simulink model "remoteMicrogrid"  (R2023a)
settings: Solver=FixedStepDiscrete  StartTime=0.0  StopTime=8  FixedStep=Ts  RelTol=1e-3
PreLoadFcn:
  | remoteMicrogridInputData
undefined symbols (not defined in the file): BESS, ControlRoom, DiscIntNeverNeededParam, Grid, Load, Machine, Microgrid, PV, T_on, Ts
libraries: ee_lib x46, eeGeneralControl x35, nesl_utility_internal x25, simulink x24, nesl_utility x20, fl_lib x17, slpidlib x12, eeTransforms x5, eeRmsMeasurement x4, eeTotalHarmonicDistorsion x4, eeSinusoidalMeasurement x3, batteryecm_lib x2
(part 1 of 5)
CloseFcn:
  | try,close(h1_remote_microgrid),end
  | clear h1_remote_microgrid
  | try,close(h2_remote_microgrid),end
  | clear h2_remote_microgrid
  | try,close(h2a_remote_microgrid),end
  | clear h2a_remote_microgrid
  | try,close(h3_remote_microgrid),end
  | clear h3_remote_microgrid
  | try,close(h4_remote_microgrid),end
  | clear h4_remote_microgrid
  | clear BESS closedLoop controller currentLoopPole
  | clear fsw_V geometricMean grid Grid inverter KI_PVPLL
  | clear KP_PVPLL logsout_remote_microgrid
  | clear Microgrid PrimaryreactancePV PrimaryresistancePV
  | clear remainingPowerPerString SecondaryreactancePV
  | clear SecondaryresistancePV sensor simlog_remote_microgrid
  | clear simulation solarPanel solarPlant TransformerPrimaryVoltagePV
  | clear TransformerRatingPV TransformerSecondaryVoltagePV
  | clear Ts Ts_V Solar logsout_remote_microgrid simlog_remote_microgrid
  | clear caseNum ControlRoom Load Machine tStart tStop
  | clear transformer_lv transformer_hv transformer_VA
  | clear transformer_winding_resistance transformer_winding_lekage_reactance
  | clear transformer_zero_sequence_reactance I_max_pu Vdc C L KV_base_new
  | clear MVA_base_new z_base n_series_cell_panel n_parallel_strings_panel
  | clear n_series_panels_per_string n_parallel_strings t_sensor
  | clear Kp_ic Ki_ic Kd Kp_v Ki_v Kd_v Vdc_base
  | clear Kp_pll Ki_pll
  | clear diode_saturation_current solar_generated_current_AM
  | clear quality_factor_i quality_factor_j Solar_cell.series_resistance
  | clear parallel_resistance temp_cofficient Eg temparature_exponent_Is1
  | clear temparature_exponent_Is2 temparature_exponent_Rs temparature_exponent_Rp
  | clear measurement_temperature device_temperature
  | clear PV Solar_cell T_on
  | clear BESSCost1 BESSCost2 BESSCost3 BESSCost4 BESSCost5 BESSKVAs1 BESSKVAs2
  | clear BESSKVAs3 BESSKVAs4 BESSKVAs5 Diesel_cost_s1 Diesel_cost_s1_yr Diesel_cost_s2
  | clear Diesel_cost_s2_yr Diesel_cost_s3 Diesel_cost_s3_yr Diesel_cost_s4 Diesel_cost_s4_yr
  | clear Diesel_cost_s5 Diesel_cost_s5_yr diesel_litre_USD Diesel_loading_100percent
  | clear Diesel_loading_25percent Diesel_loading_50percent Diesel_loading_75percent
  | clear Diesel_s1 Diesel_s2 Diesel_s3 Diesel_s4 Diesel_s5 DieselKVAs1 DieselKVAs2
  | clear DieselKVAs3 DieselKVAs4 DieselKVAs5 frequencyLimit logsout1 logsout2 logsout3
  | clear logsout4 logsout_activeloss1 logsout_activeloss2 logsout_activeloss3
  | clear logsout_activeloss4 logsout_freqmax1 logsout_freqmax2 logsout_freqmax3
  | clear logsout_freqmax4 logsout_freqmin1 logsout_freqmin2 logsout_freqmin3 logsout_freqmin4
  | clear logsout_LoadTHD1 logsout_LoadTHD2 logsout_LoadTHD3 logsout_LoadTHD4
  | clear logsout_MaxLoadVoltage1 logsout_MaxLoadVoltage2 logsout_MaxLoadVoltage3
  | clear logsout_MaxLoadVoltage4 logsout_MinLoadVoltage1 logsout_MinLoadVoltage2
  | clear logsout_MinLoadVoltage3 logsout_MinLoadVoltage4 logsout_PCCTHD1 logsout_PCCTHD2
  | clear logsout_PCCTHD3 logsout_PCCTHD4 logsout_reactiveloss1 logsout_reactiveloss2
  | clear logsout_reactiveloss3 logsout_reactiveloss4 logsout_volmax1 logsout_volmax2
  | clear logsout_volmax3 logsout_volmax4 logsout_volmin1 logsout_volmin2 logsout_volmin3
  | clear logsout_volmin4 Micorgrid TotalCost1 TotalCost2 TotalCost3 TotalCost4 TotalCost5
  | clear voltageLimit xlim xticks
Description:
  | Copyright 2022 - 2023 The MathWorks, Inc.
settings Model: Creator=The MathWorks, Inc.  LastModifiedBy=skota
settings SolverCC: AlgebraicLoopSolver=TrustRegion
settings DataIOCC: SaveOutput=off  SaveTime=off  ReturnWorkspaceOutputs=off  SignalLoggingName=logsout_remote_microgrid  OutputTimes=[0:1.1*3*Voc/(1*2000):1.1*3*Voc/1]
settings OptimizationCC: ReuseModelBlockBuffer=off
settings DebuggingCC: UnconnectedInputMsg=warning  UnconnectedOutputMsg=warning  UnconnectedLineMsg=warning  StateNameClashWarn=warning  ArithmeticOperatorsInVariantConditions=warning
settings HardwareCC: ProdBitPerPointer=32  ProdBitPerSizeT=32  ProdBitPerPtrDiffT=32  ProdWordSize=32  ProdHWDeviceType=Intel->x86-32 (Windows32)
settings ModelReferenceCC: EnableRefExpFcnMdlSchedulingChecks=on  PropagateSignalLabelsOutOfModel=off
settings SFSimCC: CustomCodeUndefinedFunction=UseInterfaceOnly
settings RTWCC: DLArmComputeVersion=19.05
settings CodeAppCC: StateflowObjectComments=on
settings SimscapeCC: SimscapeNominalValues="[{\"value\":\"1\",\"unit\":\"A\"},{\"value\":\"1\",\"unit\":\"bar\"},{\"value\":\"1\",\"unit\":\"cm^2\"},{\"value\":\"1\",\"unit\":\"cm^3/s\"},{\"value\":\"1\",\"unit\":\"kJ/kg\"},{\"value\":\"1\",\"unit\":\"kW\"},{\"value\":\"1\",\"unit\":\"l\"},{\"value\":\"1\",\"unit\":\"N\"},{\"value\":\"1\",\"unit\":\"N*m\"},{\"value\":\"1e3\",\"unit\":\"V\"}]"  SimscapeLogType=all  SimscapeLogSimulationStatistics=on  SimscapeLogName=simlog_remote_microgrid  SimscapeLogLimitData=off

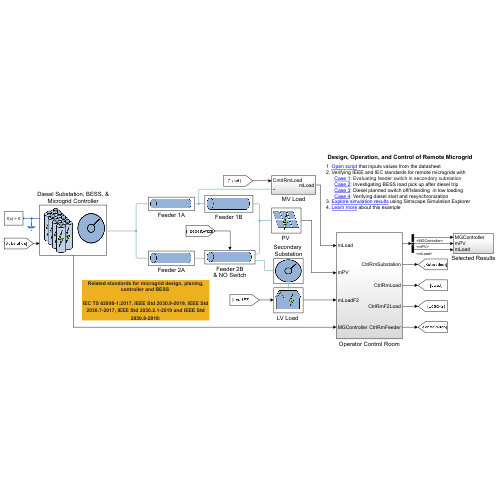
[thumbnail: Simulink's stored preview of the top-level diagram]
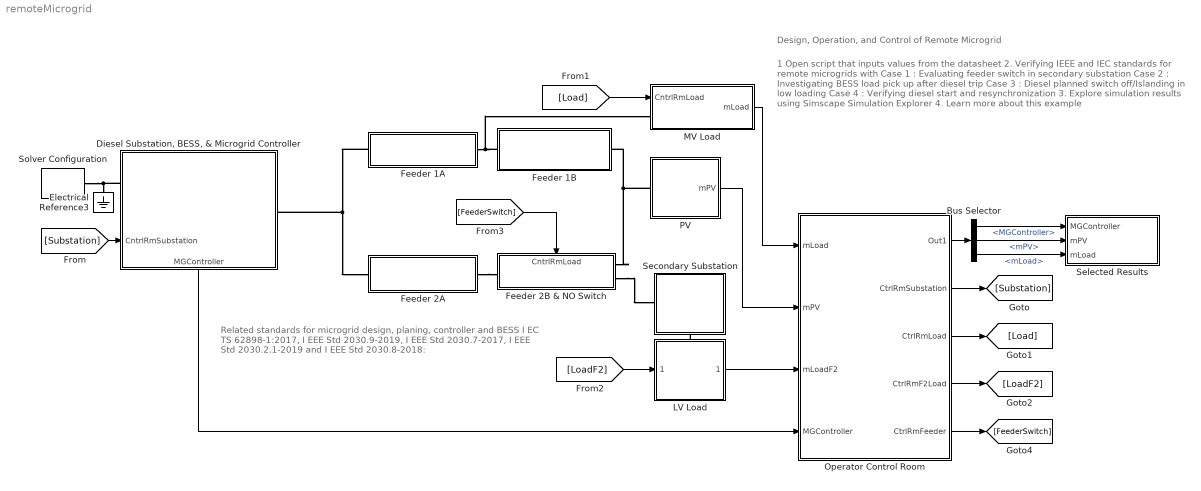
== system remoteMicrogrid ==
  note: Related standards for microgrid design, planing, controller and BESS
      | I EC TS 62898-1:2017, I EEE Std 2030.9-2019, I EEE Std 2030.7-2017, I EEE Std 2030.2.1-2019 and I EEE Std 2030.8-2018:
  note: Design, Operation, and Control of Remote Microgrid
  note: 1 Open script that inputs values from the datasheet
      | 2. Verifying IEEE and IEC standards for remote microgrids with
      | Case 1 : Evaluating feeder switch in secondary substation
      | Case 2 : Investigating BESS load pick up after diesel trip
      | Case 3 : Diesel planned switch off/Islanding in low loading
      | Case 4 : Verifying diesel start and resynchronization
      | 3. Explore simulation results using Simscape Simulation Explorer
      | 4. Learn more about this example
  Bus Selector : BusSelector  OutputSignals=MGController,mPV,mLoad
  "Diesel Substation, BESS, & Microgrid Controller" : Subsystem
      settings: PortSchema="{\"entries\":[{\"content\":{\"sides\":[{\"content\":{\"connectorIds\":[\"LConn1\",\"In1\"]},\"type\":\"ConnectorPlacement.EquallySpacedRectSide\",\"uuid\":\"34af2ba0-e960-4f27-b72f-7309cde5bec1\"},{\"content\":{\"connectorIds\":[\"RConn1\"],\"side\":\"RIGHT\"},\"type\":\"ConnectorPlacement.EquallySpacedRectSide\",\"uuid\":\"58e91d81-71e9-481c-b1fd-5cc7b2cbdd18\"},{\"content\":{\"connectorIds\":[],\"side\":\"TOP\"},\"type\":\"ConnectorPlacement.EquallySpacedRectSide\",\"uuid\":\"32e6dd42-e4bf-406e-9b62-7b4d690f744b\"},{\"content\":{\"connectorIds\":[\"Out1\"],\"side\":\"BOTTOM\"},\"type\":\"ConnectorPlacement.EquallySpacedRectSide\",\"uuid\":\"17a24731-c833-4ec2-b0a2-39897b42a00f\"}]},\"type\":\"ConnectorPlacement.EquallySpacedConnector\",\"uuid\":\"86c228e9-32f4-4f18-a8a0-642828fccfbb\"}],\"packageUris\":[\"http://schema.mathworks.com/mf0/Connector/R2020b\"],\"version\":\"1.0\"}"
      mask Display: image('$imagefile'); % Use "Edit Image" on toolstrip to change.
  Electrical Reference3 : fl_lib/Electrical/Electrical Elements/Electrical Reference
  Feeder 1A : Subsystem
      mask Display: image('$imagefile'); % Use "Edit Image" on toolstrip to change.
  Feeder 1B : Subsystem
      mask Display: image('$imagefile'); % Use "Edit Image" on toolstrip to change.
  Feeder 2A : Subsystem
      mask Display: image('$imagefile'); % Use "Edit Image" on toolstrip to change.
  Feeder 2B & NO Switch : Subsystem
      settings: PortSchema="{\"entries\":[{\"content\":{\"sides\":[{\"content\":{\"connectorIds\":[\"LConn1\"]},\"type\":\"ConnectorPlacement.EquallySpacedRectSide\",\"uuid\":\"1b47678a-34eb-4830-a1d8-8584b0b3d2f8\"},{\"content\":{\"connectorIds\":[\"RConn1\",\"RConn2\"],\"side\":\"RIGHT\"},\"type\":\"ConnectorPlacement.EquallySpacedRectSide\",\"uuid\":\"1e19bb0d-7be0-4a53-b6f3-f72359312777\"},{\"content\":{\"connectorIds\":[\"In1\"],\"side\":\"TOP\"},\"type\":\"ConnectorPlacement.EquallySpacedRectSide\",\"uuid\":\"6a5adcb0-1c8a-4af3-8ce7-b7b52f7f2199\"}]},\"type\":\"ConnectorPlacement.EquallySpacedConnector\",\"uuid\":\"0f133d9b-a960-48f9-af57-ff4de668ee2e\"}],\"packageUris\":[\"http://schema.mathworks.com/mf0/Connector/R2020b\"],\"version\":\"1.0\"}"
      mask Display: image('$imagefile'); % Use "Edit Image" on toolstrip to change.
  "LV Load " : Subsystem
      settings: PortSchema="{\"entries\":[{\"content\":{\"sides\":[{\"content\":{\"connectorIds\":[\"In1\"]},\"type\":\"ConnectorPlacement.EquallySpacedRectSide\",\"uuid\":\"cc4763ec-9449-4f2d-b299-5261ad2f5cfe\"},{\"content\":{\"connectorIds\":[\"Out1\"],\"side\":\"RIGHT\"},\"type\":\"ConnectorPlacement.EquallySpacedRectSide\",\"uuid\":\"9da329b8-70a1-4faf-a44a-2cf8be9addec\"},{\"content\":{\"connectorIds\":[\"LConn1\"],\"side\":\"TOP\"},\"type\":\"ConnectorPlacement.EquallySpacedRectSide\",\"uuid\":\"c4abe44e-3291-4dff-9d7a-9215b8ef2faf\"}]},\"type\":\"ConnectorPlacement.EquallySpacedConnector\",\"uuid\":\"e73dbaae-f88f-4a7a-af91-27ace77c935e\"}],\"packageUris\":[\"http://schema.mathworks.com/mf0/Connector/R2020b\"],\"version\":\"1.0\"}"
      mask Display: image('$imagefile'); % Use "Edit Image" on toolstrip to change.
  MV Load : Subsystem
  Operator Control Room : Subsystem
      settings: PortSchema="{\"entries\":[{\"content\":{\"sides\":[{\"content\":{\"connectorIds\":[\"Out1\",\"Out2\",\"Out3\",\"Out4\",\"Out5\"]},\"type\":\"ConnectorPlacement.EquallySpacedRectSide\",\"uuid\":\"36e3c748-e70d-4376-8c54-bee35c2cf55e\"},{\"content\":{\"connectorIds\":[\"In1\",\"In2\",\"In3\",\"In4\"],\"side\":\"RIGHT\"},\"type\":\"ConnectorPlacement.EquallySpacedRectSide\",\"uuid\":\"3af4b9ea-3351-4c6c-90c1-760bf6d2a862\"},{\"content\":{\"connectorIds\":[],\"side\":\"TOP\"},\"type\":\"ConnectorPlacement.EquallySpacedRectSide\",\"uuid\":\"c84439f5-3dbb-4f33-afb8-95498296d6fa\"}]},\"type\":\"ConnectorPlacement.EquallySpacedConnector\",\"uuid\":\"cafa6b3a-2446-4c45-9268-4fc6f6c2350c\"}],\"packageUris\":[\"http://schema.mathworks.com/mf0/Connector/R2020b\"],\"version\":\"1.0\"}"
  "PV " : Subsystem
      mask Display: image('$imagefile'); % Use "Edit Image" on toolstrip to change.
  Secondary Substation : Subsystem
      settings: PortSchema="{\"entries\":[{\"content\":{\"sides\":[{\"content\":{\"connectorIds\":[\"LConn1\"]},\"type\":\"ConnectorPlacement.EquallySpacedRectSide\",\"uuid\":\"e00206b4-f52b-4711-97fc-4887ea8823c3\"},{\"content\":{\"connectorIds\":[],\"side\":\"RIGHT\"},\"type\":\"ConnectorPlacement.EquallySpacedRectSide\",\"uuid\":\"71e01694-379b-4552-8103-40d657e486e9\"},{\"content\":{\"connectorIds\":[],\"side\":\"TOP\"},\"type\":\"ConnectorPlacement.EquallySpacedRectSide\",\"uuid\":\"04395bce-e736-431c-9f74-8350dc9d2f2b\"},{\"content\":{\"connectorIds\":[\"RConn1\"],\"side\":\"BOTTOM\"},\"type\":\"ConnectorPlacement.EquallySpacedRectSide\",\"uuid\":\"4a9ed1b9-5a03-4ea2-8ce4-b63f4eba4172\"}]},\"type\":\"ConnectorPlacement.EquallySpacedConnector\",\"uuid\":\"55927287-d52f-4d79-aceb-3e97c7a13d06\"}],\"packageUris\":[\"http://schema.mathworks.com/mf0/Connector/R2020b\"],\"version\":\"1.0\"}"
      mask Display: image('$imagefile'); % Use "Edit Image" on toolstrip to change.
  Selected Results : Subsystem
  Solver Configuration : nesl_utility_internal/Solver Configuration  PhysicalDomain=network_engine_domain  SubClassName=solver  LeftPortType=input  RightPortType=generic  Tones=[]  Harmonics=[]  SimulateNoise=off  Profile=off  UseLocalSampling=off  EnableSwitchedLinearOptims=on  FrequencyDomain=off  UseCCode=off  RelTol=0.001  AbsTol=1e-06  MinStep=1e-09  ToWorkspace=off  RevertToSquareIcSolve=off  NumHomotopyIterations=100  PhasorMode=off  PhasorModeNumHarmonics=1  ConsistencySolver=NEWTON_FTOL  IndexReductionMethod=DerivativeReplacement  DoDC=off  ResidualTolerance=1e-07  ConsistencyTolSource=GLOBAL  ConsistencyAbsTol=0.001  ConsistencyRelTol=0.001  ConsistencyTolFactor=0.001  UseLocalSolver=on  LocalSolverChoice=NE_BACKWARD_EULER_ADVANCER  ResolveIndetEquations=on  FunctionEvalNumThread=1  LocalSolverSampleTime=Ts  DoFixedCost=on  MaxNonlinIter=3  MaxModeIter=2  ComputeImpulses=off  ImpulseIterations=1  LinearAlgebra=auto  LinearAlgebraNumThread=0  EquationFormulation=NE_TIME_EF  DelaysMemoryBudget=1024  AutomaticFiltering=off  FilteringTimeConstant=0.001  PartitionStorageMethod=AS_NEEDED  PartitionMemoryBudget=1024  PartitionMethod=FAST
  wires:
  Operator Control Room/2(CtrlRmSubstation) -> [Substation]
  Bus Selector/1 -> Selected Results/1(MGController)  "<MGController>"
  Bus Selector/2 -> Selected Results/2(mPV)  "<mPV>"
  Bus Selector/3 -> Selected Results/3(mLoad)  "<mLoad>"
  Operator Control Room/1(Out1) -> Bus Selector/1
  [Substation] -> "Diesel Substation, BESS, & Microgrid Controller"/1(CntrlRmSubstation)
  "LV Load "/1(mLoadF2) -> Operator Control Room/3(mLoadF2)
  MV Load/1(mLoad) -> Operator Control Room/1(mLoad)
  "Diesel Substation, BESS, & Microgrid Controller"/1(MGController) -> Operator Control Room/4(MGController)
  [Load] -> MV Load/1(CntrlRmLoad)
  [LoadF2] -> "LV Load "/1(CtrlRmF2Load)
  Operator Control Room/3(CtrlRmLoad) -> [Load]
  Operator Control Room/4(CtrlRmF2Load) -> [LoadF2]
  Operator Control Room/5(CtrlRmFeeder) -> [FeederSwitch]
  "PV "/1(mPV) -> Operator Control Room/2(mPV)
  [FeederSwitch] -> Feeder 2B & NO Switch/1(CntrlRmLoad)
  connections:
  "LV Load "/LConn1 -- Secondary Substation/RConn1
  Solver Configuration/RConn1 -- Electrical Reference3/LConn1 -- "Diesel Substation, BESS, & Microgrid Controller"/LConn1
  "PV "/LConn1 -- Feeder 2B & NO Switch/RConn1 -- Feeder 1B/RConn1
  Feeder 1A/RConn1 -- MV Load/LConn1 -- Feeder 1B/LConn1
  Feeder 1A/LConn1 -- Feeder 2A/LConn1 -- "Diesel Substation, BESS, & Microgrid Controller"/RConn1
  Feeder 2B & NO Switch/RConn2 -- Secondary Substation/LConn1
  Feeder 2A/RConn1 -- Feeder 2B & NO Switch/LConn1

== system remoteMicrogrid/Diesel Substation, BESS, & Microgrid Controller ==
  CntrlRmSubstation : Inport
  BESS and Controller : Subsystem
  Bus Creator : BusCreator  Inputs=3
  CntrlRmSubstation1 : InportShadow
  Diesel Generator : Subsystem
  Microgrid Controller : Subsystem
      settings: PortSchema="{\"entries\":[{\"content\":{\"sides\":[{\"content\":{\"connectorIds\":[\"In1\",\"In2\",\"In3\"]},\"type\":\"ConnectorPlacement.EquallySpacedRectSide\",\"uuid\":\"5a677e32-2413-4856-9683-7f083fbde1c7\"},{\"content\":{\"connectorIds\":[\"RConn1\",\"Out1\",\"Out2\"],\"side\":\"RIGHT\"},\"type\":\"ConnectorPlacement.EquallySpacedRectSide\",\"uuid\":\"93a85587-a429-4479-a8cb-2de590d95871\"},{\"content\":{\"connectorIds\":[],\"side\":\"TOP\"},\"type\":\"ConnectorPlacement.EquallySpacedRectSide\",\"uuid\":\"c42d9fd8-4416-4e89-82a5-0d6c34ce0f8c\"}]},\"type\":\"ConnectorPlacement.EquallySpacedConnector\",\"uuid\":\"0378cbf3-df98-42a2-a108-9ea24e13e829\"}],\"packageUris\":[\"http://schema.mathworks.com/mf0/Connector/R2020b\"],\"version\":\"1.0\"}"
  PCC Measurements and PCC Breaker : Subsystem
      settings: PortSchema="{\"entries\":[{\"content\":{\"sides\":[{\"content\":{\"connectorIds\":[\"LConn1\"]},\"type\":\"ConnectorPlacement.EquallySpacedRectSide\",\"uuid\":\"04177ba8-e6a4-4482-9e4e-86e01b546ca8\"},{\"content\":{\"connectorIds\":[\"RConn1\",\"RConn2\",\"Out1\"],\"side\":\"RIGHT\"},\"type\":\"ConnectorPlacement.EquallySpacedRectSide\",\"uuid\":\"b1feeba7-b9e0-4dc8-9251-9fa4e491a467\"},{\"content\":{\"connectorIds\":[],\"side\":\"TOP\"},\"type\":\"ConnectorPlacement.EquallySpacedRectSide\",\"uuid\":\"26b7aa1a-5290-4eee-bcf5-b11865d5ca2e\"}]},\"type\":\"ConnectorPlacement.EquallySpacedConnector\",\"uuid\":\"5841c04a-e0b1-4fd8-9efd-d8c83177b337\"}],\"packageUris\":[\"http://schema.mathworks.com/mf0/Connector/R2020b\"],\"version\":\"1.0\"}"
  Transformer and Disconnectors : Subsystem
  ref : PMIOPort  Side=Left
  "~ " : PMIOPort  Port=2  Side=Right
  MGController : Outport
  wires:
  PCC Measurements and PCC Breaker/1(" mPCC") -> Microgrid Controller/1("mPCC ")
  CntrlRmSubstation/1 -> BESS and Controller/2(CntrlRmSubstation)
  BESS and Controller/1(mBESS) -> Microgrid Controller/3(BESS), Bus Creator/3  "BESS"
  Bus Creator/1 -> MGController/1
  Microgrid Controller/1(BESSRef) -> [BESSref], Bus Creator/1  "References and BRK"
  CntrlRmSubstation1/1 -> Microgrid Controller/2(CntrlRmSubstation)
  [BESSref] -> BESS and Controller/1(BESSRef)
  Microgrid Controller/2(MGController) -> Bus Creator/2  "Controller"
  connections:
  Microgrid Controller/RConn1 -- PCC Measurements and PCC Breaker/RConn2
  "~ "/RConn1 -- PCC Measurements and PCC Breaker/RConn1 -- BESS and Controller/RConn1
  Transformer and Disconnectors/RConn1 -- PCC Measurements and PCC Breaker/LConn1
  Transformer and Disconnectors/LConn1 -- Diesel Generator/RConn1
  ref/RConn1 -- Diesel Generator/LConn1

== system remoteMicrogrid/Feeder 1A ==
  "Line X/R=1.44 " : ee_lib/Passive/RLC Assemblies/RLC (Three-Phase)  component_structure=ee.enum.rlc.structure.SeriesRL  R=Microgrid.R_line Ohm  L=Microgrid.L_line H  C=1 F  R_parasitic=1e-6 Ohm  G_parasitic=1e-5 1/Ohm  IL_specify=on  IL_priority=High  IL=[0, 0, 0] A  IL_nominal_specify=off  IL_nominal_unit=A  IL_nominal_value=1  VC_specify=on  VC_priority=High  VC=[0, 0, 0] V  VC_nominal_specify=off  VC_nominal_unit=V  VC_nominal_value=1
      settings: InternalSimscapePortConfiguration="{\"Bottom\":[],\"Left\":[{\"id\":\"N1\",\"label\":\"~1\",\"type\":\"foundation.electrical.three_phase\"}],\"Right\":[{\"id\":\"N2\",\"label\":\"~2\",\"type\":\"foundation.electrical.three_phase\"}],\"Top\":[]}"
  Conn1 : PMIOPort  Side=Right
  Conn2 : PMIOPort  Port=2  Side=Left
  connections:
  "Line X/R=1.44 "/RConn1 -- Conn1/RConn1
  "Line X/R=1.44 "/LConn1 -- Conn2/RConn1

== system remoteMicrogrid/Feeder 1B ==
  Line X/R=1.44 : ee_lib/Passive/RLC Assemblies/RLC (Three-Phase)  component_structure=ee.enum.rlc.structure.SeriesRL  R=Microgrid.R_line Ohm  L=Microgrid.L_line H  C=1 F  R_parasitic=1e-6 Ohm  G_parasitic=1e-5 1/Ohm  IL_specify=on  IL_priority=High  IL=[0, 0, 0] A  IL_nominal_specify=off  IL_nominal_unit=A  IL_nominal_value=1  VC_specify=on  VC_priority=High  VC=[0, 0, 0] V  VC_nominal_specify=off  VC_nominal_unit=V  VC_nominal_value=1
      settings: InternalSimscapePortConfiguration="{\"Bottom\":[],\"Left\":[{\"id\":\"N1\",\"label\":\"~1\",\"type\":\"foundation.electrical.three_phase\"}],\"Right\":[{\"id\":\"N2\",\"label\":\"~2\",\"type\":\"foundation.electrical.three_phase\"}],\"Top\":[]}"
  Conn1 : PMIOPort  Side=Left
  Conn2 : PMIOPort  Port=2  Side=Right
  connections:
  Line X/R=1.44/LConn1 -- Conn1/RConn1
  Conn2/RConn1 -- Line X/R=1.44/RConn1

== system remoteMicrogrid/Feeder 2A ==
  "Line X/R=1.44  " : ee_lib/Passive/RLC Assemblies/RLC (Three-Phase)  component_structure=ee.enum.rlc.structure.SeriesRL  R=Microgrid.R_line Ohm  L=Microgrid.L_line H  C=1 F  R_parasitic=1e-6 Ohm  G_parasitic=1e-5 1/Ohm  IL_specify=on  IL_priority=High  IL=[0, 0, 0] A  IL_nominal_specify=off  IL_nominal_unit=A  IL_nominal_value=1  VC_specify=on  VC_priority=High  VC=[0, 0, 0] V  VC_nominal_specify=off  VC_nominal_unit=V  VC_nominal_value=1
      settings: InternalSimscapePortConfiguration="{\"Bottom\":[],\"Left\":[{\"id\":\"N1\",\"label\":\"~1\",\"type\":\"foundation.electrical.three_phase\"}],\"Right\":[{\"id\":\"N2\",\"label\":\"~2\",\"type\":\"foundation.electrical.three_phase\"}],\"Top\":[]}"
  Conn2 : PMIOPort  Side=Left
  Conn1 : PMIOPort  Port=2  Side=Right
  connections:
  Conn2/RConn1 -- "Line X/R=1.44  "/LConn1
  Conn1/RConn1 -- "Line X/R=1.44  "/RConn1

== system remoteMicrogrid/Feeder 2B & NO Switch ==
  Bus Element In2 : Inport  PortName=CntrlRmLoad  Element=FeederSwitch
  " Line X/R=1.44 " : ee_lib/Passive/RLC Assemblies/RLC (Three-Phase)  component_structure=ee.enum.rlc.structure.SeriesRL  R=Microgrid.R_line Ohm  L=Microgrid.L_line H  C=1 F  R_parasitic=1e-6 Ohm  G_parasitic=1e-5 1/Ohm  IL_specify=on  IL_priority=High  IL=[0, 0, 0] A  IL_nominal_specify=off  IL_nominal_unit=A  IL_nominal_value=1  VC_specify=on  VC_priority=High  VC=[0, 0, 0] V  VC_nominal_specify=off  VC_nominal_unit=V  VC_nominal_value=1
      settings: InternalSimscapePortConfiguration="{\"Bottom\":[],\"Left\":[{\"id\":\"N1\",\"label\":\"~1\",\"type\":\"foundation.electrical.three_phase\"}],\"Right\":[{\"id\":\"N2\",\"label\":\"~2\",\"type\":\"foundation.electrical.three_phase\"}],\"Top\":[]}"
  " Line X/R=1.44 1" : ee_lib/Passive/RLC Assemblies/RLC (Three-Phase)  component_structure=ee.enum.rlc.structure.SeriesRL  R=Microgrid.R_line Ohm  L=Microgrid.L_line H  C=1 F  R_parasitic=1e-6 Ohm  G_parasitic=1e-5 1/Ohm  IL_specify=on  IL_priority=High  IL=[0, 0, 0] A  IL_nominal_specify=off  IL_nominal_unit=A  IL_nominal_value=1  VC_specify=on  VC_priority=High  VC=[0, 0, 0] V  VC_nominal_specify=off  VC_nominal_unit=V  VC_nominal_value=1
      settings: InternalSimscapePortConfiguration="{\"Bottom\":[],\"Left\":[{\"id\":\"N1\",\"label\":\"~1\",\"type\":\"foundation.electrical.three_phase\"}],\"Right\":[{\"id\":\"N2\",\"label\":\"~2\",\"type\":\"foundation.electrical.three_phase\"}],\"Top\":[]}"
  Circuit Breaker (Three-Phase) : ee_lib/Switches & Breakers/Circuit Breaker (Three-Phase)  R_closed=0.001 Ohm  G_open=1e-6 1/Ohm  threshold=0.5 V  breaker_behavior=ee.enum.switches.breakerBehavior.zeroCrossingDisable
      settings: InternalSimscapePortConfiguration="{\"Bottom\":[],\"Left\":[{\"id\":\"vT\",\"label\":\"vT\",\"type\":\"input\"},{\"id\":\"N1\",\"label\":\"~1\",\"type\":\"foundation.electrical.three_phase\"}],\"Right\":[{\"id\":\"N2\",\"label\":\"~2\",\"type\":\"foundation.electrical.three_phase\"}],\"Top\":[]}"
  Circuit Breaker (Three-Phase)1 : ee_lib/Switches & Breakers/Circuit Breaker (Three-Phase)  R_closed=0.001 Ohm  G_open=1e-6 1/Ohm  threshold=0.5 V  breaker_behavior=ee.enum.switches.breakerBehavior.zeroCrossingDisable
      settings: InternalSimscapePortConfiguration="{\"Bottom\":[],\"Left\":[{\"id\":\"vT\",\"label\":\"vT\",\"type\":\"input\"},{\"id\":\"N1\",\"label\":\"~1\",\"type\":\"foundation.electrical.three_phase\"}],\"Right\":[{\"id\":\"N2\",\"label\":\"~2\",\"type\":\"foundation.electrical.three_phase\"}],\"Top\":[]}"
  Subsystem : Subsystem
  Conn2 : PMIOPort  Side=Left
  Feeder1BRK : PMIOPort  Port=2  Side=Right
  Feeder2BRK : PMIOPort  Port=3  Side=Right
  wires:
  Bus Element In2/1 -> Subsystem/1(ControlRoom)
  connections:
  Circuit Breaker (Three-Phase)/LConn2 -- " Line X/R=1.44 "/RConn1
  " Line X/R=1.44 1"/LConn1 -- Feeder2BRK/RConn1
  Conn2/RConn1 -- Circuit Breaker (Three-Phase)1/LConn2
  Subsystem/RConn1 -- Circuit Breaker (Three-Phase)/LConn1
  " Line X/R=1.44 "/LConn1 -- " Line X/R=1.44 1"/RConn1 -- Circuit Breaker (Three-Phase)1/RConn1
  Subsystem/RConn2 -- Circuit Breaker (Three-Phase)1/LConn1
  Circuit Breaker (Three-Phase)/RConn1 -- Feeder1BRK/RConn1

== system remoteMicrogrid/LV Load  ==
  Bus Element In3 : Inport  PortName=CtrlRmF2Load  Element=Load2BControl
  Bus Element In1 : Inport  PortName=CtrlRmF2Load  Element=Load2AControl
  Circuit Breaker (Three-Phase)1 : ee_lib/Switches & Breakers/Circuit Breaker (Three-Phase)  R_closed=0.001 Ohm  G_open=1e-6 1/Ohm  threshold=0.5 V  breaker_behavior=ee.enum.switches.breakerBehavior.zeroCrossingEnable
      settings: InternalSimscapePortConfiguration="{\"Bottom\":[],\"Left\":[{\"id\":\"vT\",\"label\":\"vT\",\"type\":\"input\"},{\"id\":\"N1\",\"label\":\"~1\",\"type\":\"foundation.electrical.three_phase\"}],\"Right\":[{\"id\":\"N2\",\"label\":\"~2\",\"type\":\"foundation.electrical.three_phase\"}],\"Top\":[]}"
  Circuit Breaker (Three-Phase)2 : ee_lib/Switches & Breakers/Circuit Breaker (Three-Phase)  R_closed=0.001 Ohm  G_open=1e-6 1/Ohm  threshold=0.5 V  breaker_behavior=ee.enum.switches.breakerBehavior.zeroCrossingEnable
      settings: InternalSimscapePortConfiguration="{\"Bottom\":[],\"Left\":[{\"id\":\"vT\",\"label\":\"vT\",\"type\":\"input\"},{\"id\":\"N1\",\"label\":\"~1\",\"type\":\"foundation.electrical.three_phase\"}],\"Right\":[{\"id\":\"N2\",\"label\":\"~2\",\"type\":\"foundation.electrical.three_phase\"}],\"Top\":[]}"
  Electrical Reference2 : fl_lib/Electrical/Electrical Elements/Electrical Reference
  Electrical Reference5 : fl_lib/Electrical/Electrical Elements/Electrical Reference
  Load Measurements1 : Subsystem
  Simulink-PS Converter1 : nesl_utility_internal/Simulink-PS Converter  PhysicalDomain=network_engine_domain  SubClassName=ps_input  LeftPortType=input  RightPortType=output  PseudoPeriodic=off  Frequencies=[]  NoiseDistribution=none  NoiseParameters=[]  Unit=1  AffineConversion=off  FilteringAndDerivatives=provide  SimscapeFilterOrder=1  InputFilterTimeConstant=0.001  UdotUserProvided=0
  Simulink-PS Converter3 : nesl_utility_internal/Simulink-PS Converter  PhysicalDomain=network_engine_domain  SubClassName=ps_input  LeftPortType=input  RightPortType=output  PseudoPeriodic=off  Frequencies=[]  NoiseDistribution=none  NoiseParameters=[]  Unit=1  AffineConversion=off  FilteringAndDerivatives=provide  SimscapeFilterOrder=1  InputFilterTimeConstant=0.001  UdotUserProvided=0
  Switchable 10 kW 480 Vrms 60 Hz : ee_lib/Passive/RLC Assemblies/Wye-Connected Load  parameterization=ee.enum.rlc.parameterization.ratedpower  component_structure=ee.enum.rlc.structure.C  component_structure_PQ=ee.enum.rlc.structure.SeriesRL  R=1 Ohm  L=0.001 H  C=1e-6 F  VRated=Microgrid.LVVoltage V  FRated=Microgrid.Frequency Hz  P=Microgrid.P_LoadF2B W  Qpos=Microgrid.Q_LoadF2B A*V  Qneg=-3000 A*V  R_parasitic=1e-6 Ohm  G_parasitic=1e-6 1/Ohm  R_parasitic_PQ=1e-6 Ohm  G_parasitic_PQ=1e-6 1/Ohm  Vmag0=Microgrid.Voltage V  Vang0=0 deg  Freq0=Microgrid.Frequency Hz  IL_specify=on  IL_priority=High  IL=[ 0 0 0 ] A  IL_nominal_specify=off  IL_nominal_unit=A  IL_nominal_value=1  VC_specify=on  VC_priority=High  VC=[ 0 0 0 ] V  VC_nominal_specify=off  VC_nominal_unit=V  VC_nominal_value=1
  Switchable 25 kW 480 Vrms 60 Hz : ee_lib/Passive/RLC Assemblies/Wye-Connected Load  parameterization=ee.enum.rlc.parameterization.ratedpower  component_structure=ee.enum.rlc.structure.C  component_structure_PQ=ee.enum.rlc.structure.SeriesRL  R=1 Ohm  L=0.001 H  C=1e-6 F  VRated=Microgrid.LVVoltage V  FRated=Microgrid.Frequency Hz  P=Microgrid.P_LoadF2A W  Qpos=Microgrid.Q_LoadF2A A*V  Qneg=-3000 A*V  R_parasitic=1e-6 Ohm  G_parasitic=1e-6 1/Ohm  R_parasitic_PQ=1e-6 Ohm  G_parasitic_PQ=1e-6 1/Ohm  Vmag0=Microgrid.Voltage V  Vang0=0 deg  Freq0=Microgrid.Frequency Hz  IL_specify=on  IL_priority=High  IL=[ 0 0 0 ] A  IL_nominal_specify=off  IL_nominal_unit=A  IL_nominal_value=1  VC_specify=on  VC_priority=High  VC=[ 0 0 0 ] V  VC_nominal_specify=off  VC_nominal_unit=V  VC_nominal_value=1
  ~ : PMIOPort  Side=Left
  mLoadF2 : Outport
  wires:
  Load Measurements1/1(mLoadF2) -> mLoadF2/1
  Bus Element In1/1 -> Simulink-PS Converter3/1
  Bus Element In3/1 -> Simulink-PS Converter1/1
  connections:
  Electrical Reference2/LConn1 -- Switchable 25 kW 480 Vrms 60 Hz/RConn1
  Simulink-PS Converter3/RConn1 -- Circuit Breaker (Three-Phase)1/LConn1
  Simulink-PS Converter1/RConn1 -- Circuit Breaker (Three-Phase)2/LConn1
  ~/RConn1 -- Load Measurements1/LConn1
  Circuit Breaker (Three-Phase)1/RConn1 -- Switchable 25 kW 480 Vrms 60 Hz/LConn1
  Switchable 10 kW 480 Vrms 60 Hz/LConn1 -- Circuit Breaker (Three-Phase)2/RConn1
  Switchable 10 kW 480 Vrms 60 Hz/RConn1 -- Electrical Reference5/LConn1
  Load Measurements1/RConn1 -- Circuit Breaker (Three-Phase)2/LConn2 -- Circuit Breaker (Three-Phase)1/LConn2

== system remoteMicrogrid/MV Load ==
  Bus Element In3 : Inport  PortName=CntrlRmLoad  Element=Load2Control
  Bus Element In1 : Inport  PortName=CntrlRmLoad  Element=Load1Control
  Circuit Breaker (Three-Phase)1 : ee_lib/Switches & Breakers/Circuit Breaker (Three-Phase)  R_closed=0.001 Ohm  G_open=1e-6 1/Ohm  threshold=0.5 V  breaker_behavior=ee.enum.switches.breakerBehavior.zeroCrossingEnable
      settings: InternalSimscapePortConfiguration="{\"Bottom\":[],\"Left\":[{\"id\":\"vT\",\"label\":\"vT\",\"type\":\"input\"},{\"id\":\"N1\",\"label\":\"~1\",\"type\":\"foundation.electrical.three_phase\"}],\"Right\":[{\"id\":\"N2\",\"label\":\"~2\",\"type\":\"foundation.electrical.three_phase\"}],\"Top\":[]}"
  Circuit Breaker (Three-Phase)2 : ee_lib/Switches & Breakers/Circuit Breaker (Three-Phase)  R_closed=0.001 Ohm  G_open=1e-6 1/Ohm  threshold=0.5 V  breaker_behavior=ee.enum.switches.breakerBehavior.zeroCrossingEnable
      settings: InternalSimscapePortConfiguration="{\"Bottom\":[],\"Left\":[{\"id\":\"vT\",\"label\":\"vT\",\"type\":\"input\"},{\"id\":\"N1\",\"label\":\"~1\",\"type\":\"foundation.electrical.three_phase\"}],\"Right\":[{\"id\":\"N2\",\"label\":\"~2\",\"type\":\"foundation.electrical.three_phase\"}],\"Top\":[]}"
  Electrical Reference2 : fl_lib/Electrical/Electrical Elements/Electrical Reference
  Electrical Reference5 : fl_lib/Electrical/Electrical Elements/Electrical Reference
  Load Measurements1 : Subsystem
  Simulink-PS Converter1 : nesl_utility_internal/Simulink-PS Converter  PhysicalDomain=network_engine_domain  SubClassName=ps_input  LeftPortType=input  RightPortType=output  PseudoPeriodic=off  Frequencies=[]  NoiseDistribution=none  NoiseParameters=[]  Unit=1  AffineConversion=off  FilteringAndDerivatives=provide  SimscapeFilterOrder=1  InputFilterTimeConstant=0.001  UdotUserProvided=0
  Simulink-PS Converter3 : nesl_utility_internal/Simulink-PS Converter  PhysicalDomain=network_engine_domain  SubClassName=ps_input  LeftPortType=input  RightPortType=output  PseudoPeriodic=off  Frequencies=[]  NoiseDistribution=none  NoiseParameters=[]  Unit=1  AffineConversion=off  FilteringAndDerivatives=provide  SimscapeFilterOrder=1  InputFilterTimeConstant=0.001  UdotUserProvided=0
  Switchable 115 kW 4160 Vrms 60 Hz : ee_lib/Passive/RLC Assemblies/Wye-Connected Load  parameterization=ee.enum.rlc.parameterization.ratedpower  component_structure=ee.enum.rlc.structure.C  component_structure_PQ=ee.enum.rlc.structure.SeriesRL  R=1 Ohm  L=0.001 H  C=1e-6 F  VRated=Microgrid.Voltage V  FRated=Microgrid.Frequency Hz  P=Microgrid.P_LoadF1A W  Qpos=Microgrid.Q_LoadF1A A*V  Qneg=-3000 A*V  R_parasitic=1e-6 Ohm  G_parasitic=1e-6 1/Ohm  R_parasitic_PQ=1e-6 Ohm  G_parasitic_PQ=1e-6 1/Ohm  Vmag0=Microgrid.Voltage V  Vang0=0 deg  Freq0=Microgrid.Frequency Hz  IL_specify=on  IL_priority=High  IL=[ 0 0 0 ] A  IL_nominal_specify=off  IL_nominal_unit=A  IL_nominal_value=1  VC_specify=on  VC_priority=High  VC=[ 0 0 0 ] V  VC_nominal_specify=off  VC_nominal_unit=V  VC_nominal_value=1
  Switchable 30 kW 4160 Vrms 60 Hz1 : ee_lib/Passive/RLC Assemblies/Wye-Connected Load  parameterization=ee.enum.rlc.parameterization.ratedpower  component_structure=ee.enum.rlc.structure.C  component_structure_PQ=ee.enum.rlc.structure.SeriesRL  R=1 Ohm  L=0.001 H  C=1e-6 F  VRated=Microgrid.Voltage V  FRated=Microgrid.Frequency Hz  P=Microgrid.P_LoadF1B W  Qpos=Microgrid.Q_LoadF1B A*V  Qneg=-3000 A*V  R_parasitic=1e-6 Ohm  G_parasitic=1e-6 1/Ohm  R_parasitic_PQ=1e-6 Ohm  G_parasitic_PQ=1e-6 1/Ohm  Vmag0=Microgrid.Voltage V  Vang0=0 deg  Freq0=Microgrid.Frequency Hz  IL_specify=on  IL_priority=High  IL=[ 0 0 0 ] A  IL_nominal_specify=off  IL_nominal_unit=A  IL_nominal_value=1  VC_specify=on  VC_priority=High  VC=[ 0 0 0 ] V  VC_nominal_specify=off  VC_nominal_unit=V  VC_nominal_value=1
  ~ : PMIOPort  Side=Left
  mLoad : Outport
  wires:
  Bus Element In3/1 -> Simulink-PS Converter1/1
  Bus Element In1/1 -> Simulink-PS Converter3/1
  Load Measurements1/1(mLoad) -> mLoad/1
  connections:
  Switchable 30 kW 4160 Vrms 60 Hz1/RConn1 -- Electrical Reference5/LConn1
  Switchable 30 kW 4160 Vrms 60 Hz1/LConn1 -- Circuit Breaker (Three-Phase)2/RConn1
  Circuit Breaker (Three-Phase)1/RConn1 -- Switchable 115 kW 4160 Vrms 60 Hz/LConn1
  ~/RConn1 -- Load Measurements1/LConn1
  Simulink-PS Converter1/RConn1 -- Circuit Breaker (Three-Phase)2/LConn1
  Circuit Breaker (Three-Phase)1/LConn2 -- Circuit Breaker (Three-Phase)2/LConn2 -- Load Measurements1/RConn1
  Simulink-PS Converter3/RConn1 -- Circuit Breaker (Three-Phase)1/LConn1
  Electrical Reference2/LConn1 -- Switchable 115 kW 4160 Vrms 60 Hz/RConn1

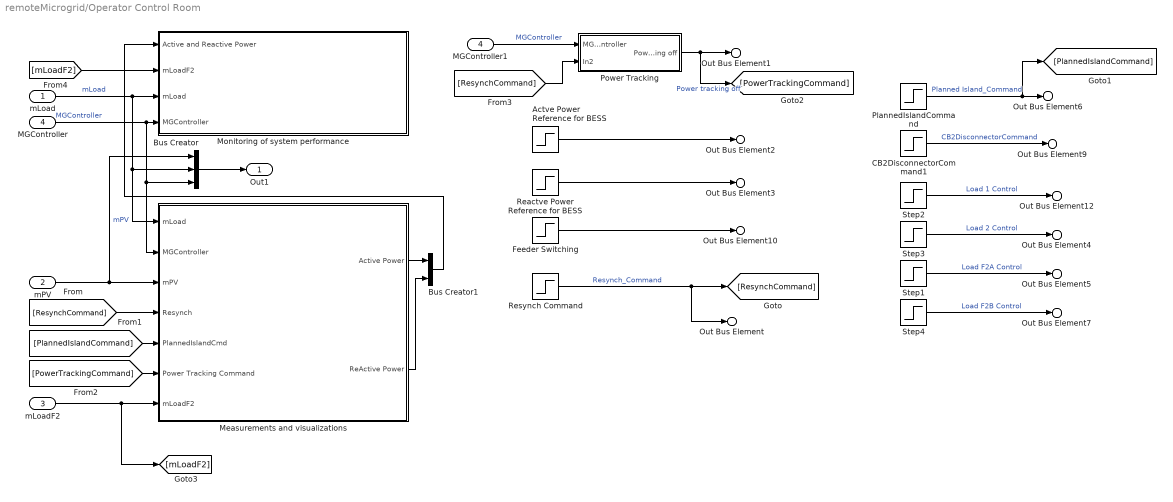
== system remoteMicrogrid/Operator Control Room ==
  mLoad : Inport
  mPV : Inport  Port=2
  mLoadF2 : Inport  Port=3
  MGController : Inport  Port=4
  Actve Power Reference for BESS : Step  Time=50  Before=BESS.Pref  SampleTime=Ts
  Bus Creator : BusCreator  Inputs=3
  Bus Creator1 : BusCreator  Inputs=2
  CB2DisconnectorCommand1 : Step  Time=ControlRoom.BRKControl  SampleTime=Ts
  Feeder Switching : Step  Time=ControlRoom.FeederSwitchTime  SampleTime=Ts
  MGController1 : InportShadow  Port=4
  "Measurements and visualizations " : Subsystem
  Monitoring of system performance : Subsystem
  PlannedIslandCommand : Step  Time=ControlRoom.PlannedIsland  SampleTime=Ts
  Power Tracking : Subsystem
  Reactve Power Reference for BESS : Step  Time=80  Before=BESS.Qref  After=BESS.Qref  SampleTime=Ts
  Resynch Command : Step  Time=ControlRoom.Resynch  SampleTime=Ts
  Step1 : Step  Time=Load.F2AControl  SampleTime=Ts
  Step2 : Step  Time=Load.F1AControl  SampleTime=Ts
  Step3 : Step  Time=Load.F1BControl  SampleTime=Ts
  Step4 : Step  Time=Load.F2BControl  SampleTime=Ts
  Out1 : Outport
  Out Bus Element2 : Outport  Port=2  PortName=CtrlRmSubstation  Element=Pref
  Out Bus Element3 : Outport  Port=2  PortName=CtrlRmSubstation  Element=Qref
  Out Bus Element9 : Outport  Port=2  PortName=CtrlRmSubstation  Element=BRKcontrol
  Out Bus Element6 : Outport  Port=2  PortName=CtrlRmSubstation  Element=PlannedIslandCmd
  Out Bus Element : Outport  Port=2  PortName=CtrlRmSubstation  Element=ResynchCmd
  Out Bus Element1 : Outport  Port=2  PortName=CtrlRmSubstation  Element=PowerCmd
  Out Bus Element12 : Outport  Port=3  PortName=CtrlRmLoad  Element=Load1Control
  Out Bus Element4 : Outport  Port=3  PortName=CtrlRmLoad  Element=Load2Control
  Out Bus Element5 : Outport  Port=4  PortName=CtrlRmF2Load  Element=Load2AControl
  Out Bus Element7 : Outport  Port=4  PortName=CtrlRmF2Load  Element=Load2BControl
  Out Bus Element10 : Outport  Port=5  PortName=CtrlRmFeeder  Element=FeederSwitch
  wires:
  Step2/1 -> Out Bus Element12/1  "Load 1 Control"
  Step3/1 -> Out Bus Element4/1  "Load 2 Control"
  MGController/1 -> "Measurements and visualizations "/2(MGController), Bus Creator/3, Monitoring of system performance/4(MGController)  "MGController"
  [ResynchCommand] -> "Measurements and visualizations "/4(Resynch)
  mLoad/1 -> "Measurements and visualizations "/1(mLoad), Bus Creator/2, Monitoring of system performance/3(mLoad)  "mLoad"
  CB2DisconnectorCommand1/1 -> Out Bus Element9/1  "CB2DisconnectorCommand"
  mPV/1 -> Bus Creator/1, "Measurements and visualizations "/3(mPV)  "mPV"
  PlannedIslandCommand/1 -> [PlannedIslandCommand], Out Bus Element6/1  "Planned Island_Command"
  [PlannedIslandCommand] -> "Measurements and visualizations "/5(PlannedIslandCmd)
  [PowerTrackingCommand] -> "Measurements and visualizations "/6(Power Tracking Command)
  Actve Power Reference for BESS/1 -> Out Bus Element2/1
  Reactve Power Reference for BESS/1 -> Out Bus Element3/1
  Step1/1 -> Out Bus Element5/1  "Load F2A Control"
  Step4/1 -> Out Bus Element7/1  "Load F2B Control"
  mLoadF2/1 -> [mLoadF2], "Measurements and visualizations "/7(mLoadF2)
  MGController1/1 -> Power Tracking/1(MGController)  "MGController"
  Resynch Command/1 -> Out Bus Element/1, [ResynchCommand]  "Resynch_Command"
  Power Tracking/1(Power tracking off) -> [PowerTrackingCommand], Out Bus Element1/1  "Power tracking off"
  [ResynchCommand] -> Power Tracking/2(In2)
  Feeder Switching/1 -> Out Bus Element10/1
  Bus Creator/1 -> Out1/1
  "Measurements and visualizations "/1(Active Power) -> Bus Creator1/1
  "Measurements and visualizations "/2(ReActive Power) -> Bus Creator1/2
  Bus Creator1/1 -> Monitoring of system performance/1(Active and Reactive Power)
  [mLoadF2] -> Monitoring of system performance/2(mLoadF2)

== system remoteMicrogrid/PV  ==
  30 kW PV : Subsystem
      settings: PortSchema="{\"entries\":[{\"content\":{\"sides\":[{\"content\":{\"connectorIds\":[\"Out1\",\"In1\",\"LConn1\"]},\"type\":\"ConnectorPlacement.EquallySpacedRectSide\",\"uuid\":\"cc4763ec-9449-4f2d-b299-5261ad2f5cfe\"},{\"content\":{\"connectorIds\":[],\"side\":\"RIGHT\"},\"type\":\"ConnectorPlacement.EquallySpacedRectSide\",\"uuid\":\"9da329b8-70a1-4faf-a44a-2cf8be9addec\"},{\"content\":{\"connectorIds\":[],\"side\":\"TOP\"},\"type\":\"ConnectorPlacement.EquallySpacedRectSide\",\"uuid\":\"c4abe44e-3291-4dff-9d7a-9215b8ef2faf\"}]},\"type\":\"ConnectorPlacement.EquallySpacedConnector\",\"uuid\":\"e73dbaae-f88f-4a7a-af91-27ace77c935e\"}],\"packageUris\":[\"http://schema.mathworks.com/mf0/Connector/R2020b\"],\"version\":\"1.0\"}"
  415 V/ 4.16 kV : ee_lib/Passive/Transformers/Two-Winding Transformer (Three-Phase)  SRated=PV.transformer_VA A*V  FRated=Grid.Frequency Hz  Winding1Connection=ee.enum.windingconnection.Yg  VRated1=PV.transformer_hv V  Winding2Connection=ee.enum.windingconnection.Yn  VRated2=PV.transformer_lv V  CoreType=ee.enum.coretype.threelimb  pu_Rw1=PV.transformer_winding_resistance/2  pu_Rw2=PV.transformer_winding_resistance/2  leakage_reactance_option=ee.enum.transformer_leakage.include  pu_Xl1=PV.transformer_winding_lekage_reactance/2  pu_Xl2=PV.transformer_winding_lekage_reactance/2  magnetizing_resistance_option=ee.enum.transformer_magnetizingResistance.exclude  pu_Rm=500  magnetizing_reactance_option=ee.enum.transformer_magnetizingReactance.exclude  saturation_option=ee.enum.transformer_saturation.exclude  pu_Xm=500  current_data=[0, .002, 1, 2]  magnetic_flux_data=[0, 1.2, 1.5, 1.51]  pu_X0=PV.transformer_zero_sequence_reactance  i1_specify=off  i1_priority=None  i1=[0, 0, 0] A  i1_nominal_specify=off  i1_nominal_unit=A  i1_nominal_value=1  i2_specify=off  i2_priority=None  i2=[0, 0, 0] A  i2_nominal_specify=off  i2_nominal_unit=A  i2_nominal_value=1  phi_specify=off  phi_priority=None  phi=[0, 0, 0]  phi_nominal_specify=off  phi_nominal_unit=1  phi_nominal_value=1  power_dissipated_specify=off  power_dissipated_priority=None  power_dissipated=0 W  power_dissipated_nominal_specify=off  power_dissipated_nominal_unit=W  power_dissipated_nominal_value=1
      settings: InternalSimscapePortConfiguration="{\"Bottom\":[],\"Left\":[{\"id\":\"N1\",\"label\":\"~1\",\"type\":\"foundation.electrical.three_phase\"}],\"Right\":[{\"id\":\"N2\",\"label\":\"~2\",\"type\":\"foundation.electrical.three_phase\"},{\"id\":\"n2\",\"label\":\"n2\",\"type\":\"foundation.electrical.electrical\"}],\"Top\":[]}"
  Bus Creator : BusCreator  Inputs=3
  Bus Creator1 : BusCreator  Inputs=2
  Current and Voltage Sensor (Three-Phase)5 : ee_lib/Sensors & Transducers/Current and Voltage Sensor (Three-Phase)  vMeasurementType=ee.enum.vmeasurement.lg  outputUnit=ee.enum.unit.pu  SRated=PV.MVA_base_new A*V  VRated=PV.KV_base_new V  I_specify=off  I_priority=None  I=[0, 0, 0] A  I_nominal_specify=off  I_nominal_unit=A  I_nominal_value=1  V_specify=off  V_priority=None  V=[0, 0, 0] V  V_nominal_specify=off  V_nominal_unit=V  V_nominal_value=1
      settings: InternalSimscapePortConfiguration="{\"Bottom\":[],\"Left\":[{\"id\":\"N1\",\"label\":\"~1\",\"type\":\"foundation.electrical.three_phase\"}],\"Right\":[{\"id\":\"V_output\",\"label\":\"V\",\"type\":\"output\"},{\"id\":\"I_output\",\"label\":\"I\",\"type\":\"output\"},{\"id\":\"N2\",\"label\":\"~2\",\"type\":\"foundation.electrical.three_phase\"}],\"Top\":[]}"
  Electrical Reference8 : fl_lib/Electrical/Electrical Elements/Electrical Reference
  PLL & Measurements : Subsystem
      settings: PortSchema="{\"entries\":[{\"content\":{\"sides\":[{\"content\":{\"connectorIds\":[\"Out1\",\"In1\"]},\"type\":\"ConnectorPlacement.EquallySpacedRectSide\",\"uuid\":\"76485780-20fe-4fcf-8224-69648da6ed2a\"},{\"content\":{\"connectorIds\":[],\"side\":\"RIGHT\"},\"type\":\"ConnectorPlacement.EquallySpacedRectSide\",\"uuid\":\"f19a6390-e634-42c7-8d46-4cd80cbab182\"},{\"content\":{\"connectorIds\":[],\"side\":\"TOP\"},\"type\":\"ConnectorPlacement.EquallySpacedRectSide\",\"uuid\":\"87682f72-1844-428e-be70-ad7ca3191ee3\"}]},\"type\":\"ConnectorPlacement.EquallySpacedConnector\",\"uuid\":\"f2136b07-48ec-402b-adb3-18c0bac2157c\"}],\"packageUris\":[\"http://schema.mathworks.com/mf0/Connector/R2020b\"],\"version\":\"1.0\"}"
  PS-Simulink Converter1 : nesl_utility/PS-Simulink Converter  PhysicalDomain=network_engine_domain  SubClassName=ps_output  LeftPortType=input  RightPortType=output  PseudoPeriodic=off  Frequencies=[]  VectorFormat=inherit  Unit=inherit  AffineConversion=off
  PS-Simulink Converter2 : nesl_utility/PS-Simulink Converter  PhysicalDomain=network_engine_domain  SubClassName=ps_output  LeftPortType=input  RightPortType=output  PseudoPeriodic=off  Frequencies=[]  VectorFormat=inherit  Unit=inherit  AffineConversion=off
  ~ : PMIOPort  Side=Left
  mPV : Outport
  wires:
  PS-Simulink Converter2/1 -> Bus Creator1/1, PLL & Measurements/1(V)  "Va"
  PLL & Measurements/1(PV) -> Bus Creator/2, 30 kW PV/1(PV)  "PV voltage"
  30 kW PV/1(PV power) -> Bus Creator/1  "PV power"
  Bus Creator/1 -> mPV/1
  PS-Simulink Converter1/1 -> Bus Creator1/2  "Ia"
  Bus Creator1/1 -> Bus Creator/3  "PV ac"
  connections:
  Electrical Reference8/LConn1 -- 415 V/ 4.16 kV/RConn2
  ~/RConn1 -- 415 V/ 4.16 kV/LConn1
  30 kW PV/LConn1 -- Current and Voltage Sensor (Three-Phase)5/LConn1
  415 V/ 4.16 kV/RConn1 -- Current and Voltage Sensor (Three-Phase)5/RConn3
  PS-Simulink Converter2/LConn1 -- Current and Voltage Sensor (Three-Phase)5/RConn1
  Current and Voltage Sensor (Three-Phase)5/RConn2 -- PS-Simulink Converter1/LConn1

== system remoteMicrogrid/Secondary Substation ==
  Two-Winding Transformer (Three-Phase)1 : ee_lib/Passive/Transformers/Two-Winding Transformer (Three-Phase)  SRated=Microgrid.LVLoadTransformerRating A*V  FRated=Grid.Frequency Hz  Winding1Connection=ee.enum.windingconnection.Y  VRated1=Microgrid.LVLoadTransformerPrimaryRating V  Winding2Connection=ee.enum.windingconnection.Y  VRated2=Microgrid.LVLoadTransformerSecondaryRating V  CoreType=ee.enum.coretype.threelimb  pu_Rw1=Grid.Primaryresistance  pu_Rw2=Grid.Primaryreactance  leakage_reactance_option=ee.enum.transformer_leakage.include  pu_Xl1=Grid.Secondaryresistance  pu_Xl2=Grid.Secondaryreactance  magnetizing_resistance_option=ee.enum.transformer_magnetizingResistance.include  pu_Rm=500  magnetizing_reactance_option=ee.enum.transformer_magnetizingReactance.include  saturation_option=ee.enum.transformer_saturation.exclude  pu_Xm=500  current_data=[0, .002, 1, 2]  magnetic_flux_data=[0, 1.2, 1.5, 1.51]  pu_X0=0.5  i1_specify=on  i1_priority=None  i1=[0, 0, 0] A  i1_nominal_specify=off  i1_nominal_unit=A  i1_nominal_value=1  i2_specify=on  i2_priority=None  i2=[0, 0, 0] A  i2_nominal_specify=off  i2_nominal_unit=A  i2_nominal_value=1  phi_specify=off  phi_priority=None  phi=[0, 0, 0]  phi_nominal_specify=off  phi_nominal_unit=1  phi_nominal_value=1  power_dissipated_specify=off  power_dissipated_priority=None  power_dissipated=0 W  power_dissipated_nominal_specify=off  power_dissipated_nominal_unit=W  power_dissipated_nominal_value=1
      settings: InternalSimscapePortConfiguration="{\"Bottom\":[],\"Left\":[{\"id\":\"N1\",\"label\":\"~1\",\"type\":\"foundation.electrical.three_phase\"}],\"Right\":[{\"id\":\"N2\",\"label\":\"~2\",\"type\":\"foundation.electrical.three_phase\"}],\"Top\":[]}"
  "~ " : PMIOPort  Side=Left
  ~ : PMIOPort  Port=2  Side=Right
  connections:
  Two-Winding Transformer (Three-Phase)1/RConn1 -- ~/RConn1
  "~ "/RConn1 -- Two-Winding Transformer (Three-Phase)1/LConn1

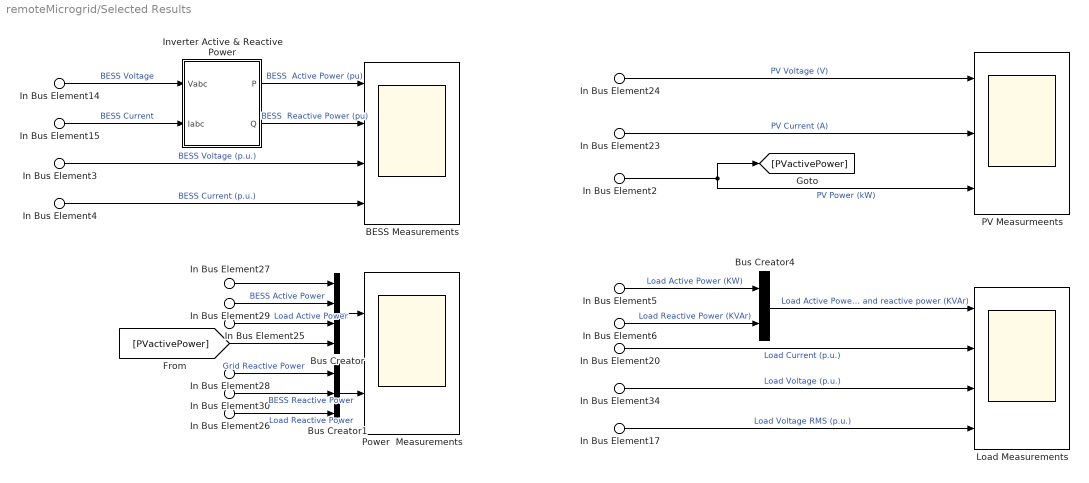
== system remoteMicrogrid/Selected Results ==
  In Bus Element27 : Inport  PortName=MGController  Element=Controller.ResynchMGController.PCC measurments.PCC.mPCC.activepower
  In Bus Element28 : Inport  PortName=MGController  Element=Controller.ResynchMGController.PCC measurments.PCC.mPCC.reactivepower
  In Bus Element14 : Inport  PortName=MGController  Element=BESS.voltage
  In Bus Element3 : Inport  PortName=MGController  Element=BESS.voltage
  In Bus Element15 : Inport  PortName=MGController  Element=BESS.current
  In Bus Element4 : Inport  PortName=MGController  Element=BESS.current
  In Bus Element29 : Inport  PortName=MGController  Element=BESS.active power
  In Bus Element30 : Inport  PortName=MGController  Element=BESS.reactive power
  In Bus Element2 : Inport  Port=2  PortName=mPV  Element=PV power.PV active power
  In Bus Element24 : Inport  Port=2  PortName=mPV  Element=PV ac.Va
  In Bus Element23 : Inport  Port=2  PortName=mPV  Element=PV ac.Ia
  In Bus Element25 : Inport  Port=3  PortName=mLoad  Element=active power
  In Bus Element5 : Inport  Port=3  PortName=mLoad  Element=active power
  In Bus Element17 : Inport  Port=3  PortName=mLoad  Element=voltageRMS
  In Bus Element20 : Inport  Port=3  PortName=mLoad  Element=current
  In Bus Element26 : Inport  Port=3  PortName=mLoad  Element=reactive power
  In Bus Element6 : Inport  Port=3  PortName=mLoad  Element=reactive power
  In Bus Element34 : Inport  Port=3  PortName=mLoad  Element=voltage
  BESS Measurements : Scope  NumInputPorts=4
  Bus Creator : BusCreator  Inputs=4
  Bus Creator1 : BusCreator  Inputs=3
  Bus Creator4 : BusCreator  Inputs=2
  "Inverter Active & Reactive Power " : Subsystem
  Load Measurements : Scope  NumInputPorts=4
  PV Measurmeents : Scope  NumInputPorts=3
  Power  Measurements : Scope  NumInputPorts=2
  wires:
  In Bus Element29/1 -> Bus Creator/2  "BESS Active Power"
  In Bus Element30/1 -> Bus Creator1/2  "BESS Reactive Power"
  In Bus Element14/1 -> "Inverter Active & Reactive Power "/1(Vabc)  "BESS Voltage"
  In Bus Element25/1 -> Bus Creator/3  "Load Active Power"
  In Bus Element20/1 -> Load Measurements/2  "Load Current (p.u.)"
  In Bus Element15/1 -> "Inverter Active & Reactive Power "/2(Iabc)  "BESS Current"
  In Bus Element28/1 -> Bus Creator1/1  "Grid Reactive Power"
  In Bus Element26/1 -> Bus Creator1/3  "Load Reactive Power"
  In Bus Element17/1 -> Load Measurements/4  "Load Voltage RMS (p.u.)"
  "Inverter Active & Reactive Power "/1(P) -> BESS Measurements/1  "BESS  Active Power (pu)"
  In Bus Element2/1 -> PV Measurmeents/3, [PVactivePower]  "PV Power (kW)"
  "Inverter Active & Reactive Power "/2(Q) -> BESS Measurements/2  "BESS  Reactive Power (pu)"
  Bus Creator/1 -> Power  Measurements/1
  In Bus Element27/1 -> Bus Creator/1
  Bus Creator1/1 -> Power  Measurements/2
  [PVactivePower] -> Bus Creator/4
  In Bus Element5/1 -> Bus Creator4/1  "Load Active Power (KW)"
  In Bus Element6/1 -> Bus Creator4/2  "Load Reactive Power (KVAr)"
  Bus Creator4/1 -> Load Measurements/1  "Load Active Power (kW) and reactive power (KVAr)"
  In Bus Element3/1 -> BESS Measurements/3  "BESS Voltage (p.u.)"
  In Bus Element4/1 -> BESS Measurements/4  "BESS Current (p.u.)"
  In Bus Element34/1 -> Load Measurements/3  "Load Voltage (p.u.)"
  In Bus Element24/1 -> PV Measurmeents/1  "PV Voltage (V)"
  In Bus Element23/1 -> PV Measurmeents/2  "PV Current (A)"

== system remoteMicrogrid/Diesel Substation, BESS, & Microgrid Controller/BESS and Controller ==
  In Bus Element34 : Inport  PortName=BESSRef  Element=Frequency
  In Bus Element1 : Inport  PortName=BESSRef  Element=Voltage
  In Bus Element2 : Inport  PortName=BESSRef  Element=Power
  CntrlRmSubstation : Inport  Port=2
  BESS : Subsystem
  BESS Control : Subsystem  mask{Kp_P=BESS.Kp_P, Ki_P=BESS.Ki_P, Kp_Q=BESS.Kp_Q, Ki_Q=BESS.Ki_Q, Kp_vd=BESS.Kp_vd, Ki_vd=BESS.Ki_vd, Kp_vq=BESS.Kp_vq, Ki_vq=BESS.Ki_vq}
      mask prompts: Kp_P "Active power tracking proportional gain"; Ki_P "Active power tracking integral gain"; Kp_Q "Reactive power tracking proportional gain"; Ki_Q "Reactive power tracking integral gain"; Kp_vd "d axis voltage controller proportional gain"; Ki_vd "d axis voltage controller integral gain"; Kp_vq "q axis voltage controller proportional gain"; Ki_vq "q axis voltage controller integral gain"
  "BESS Converter Measurement " : Subsystem
  BESS Output Filter and Transformer : Subsystem
  ~ : PMIOPort  Side=Right
  mBESS : Outport
  wires:
  In Bus Element34/1 -> BESS Control/2(f0)
  In Bus Element1/1 -> BESS Control/3(Vref)
  CntrlRmSubstation/1 -> BESS Control/4(CntrlRmSubstation)
  "BESS Converter Measurement "/1(mBESS) -> BESS Control/1(mBESS), mBESS/1
  In Bus Element2/1 -> BESS Control/5(PQref)
  connections:
  "BESS Converter Measurement "/LConn1 -- BESS Output Filter and Transformer/RConn1
  BESS Control/RConn1 -- BESS/LConn1
  BESS/LConn2 -- BESS Output Filter and Transformer/LConn1
  "BESS Converter Measurement "/RConn1 -- ~/RConn1
